simulink model "P1"  (R2020b)
settings: Solver=VariableStepAuto  StartTime=0.0  StopTime=10  RelTol=1e-3
libraries: simulink x1
settings Model: Creator=cesar  LastModifiedBy=cesar

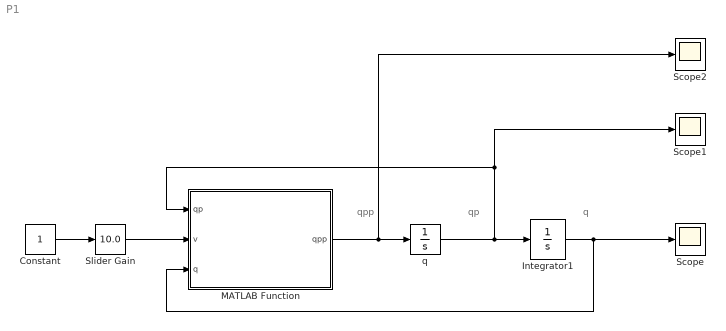
== system P1 ==
  note: qpp
  note: qp
  note: q
  Constant : Constant
  Integrator1 : Integrator  InitialCondition=1
  MATLAB Function : MATLAB Function  TreatAsAtomicUnit=on
  Scope : Scope
  Scope1 : Scope
  Scope2 : Scope
  Slider Gain : simulink/Math Operations/Slider Gain  gain=10.0  low=0  high=10
  q : Integrator  InitialCondition=1
  wires:
  MATLAB Function/1(qpp) -> q/1, Scope2/1
  q/1 -> Scope1/1, MATLAB Function/1(qp), Integrator1/1
  Integrator1/1 -> Scope/1, MATLAB Function/3(q)
  Constant/1 -> Slider Gain/1
  Slider Gain/1 -> MATLAB Function/2(v)

== matlab function P1/MATLAB Function ==
  data: qpp output; qp input; v input; q input
function qpp = pendulo(qp, v, q)
%Valores de los parámetros del sistema
g=9.81;
Jm=5;
m=5;
J=5;
l=1;
JL=J+m*l^2;
lb=0.5;
r=1;
fm=1;
fL=0.5;
Ka=1;
Kb=30;
Ra=1;
mb=1;
KL=((mb*lb)+(m*l))*g;
%Ecuación del modelo dinámico
qpp= - ((fm + fL/r^2 + (Ka*Kb)/Ra)/(Jm+(JL*r^2)))*qp - ...
       ((KL/r^2)*sin(q))/(Jm+(JL*r^2)) + ...
       ((Ka/r*Ra)/(Jm+(JL*r^2)))*v;
